simulink model "sampleModel1895"  (R2023a)
settings: Solver=VariableStepAuto  StartTime=0.0  StopTime=10.0  RelTol=1e-3
libraries: hdlsllib x3, simulink x1
settings Model: Creator=user1  LastModifiedBy=user1

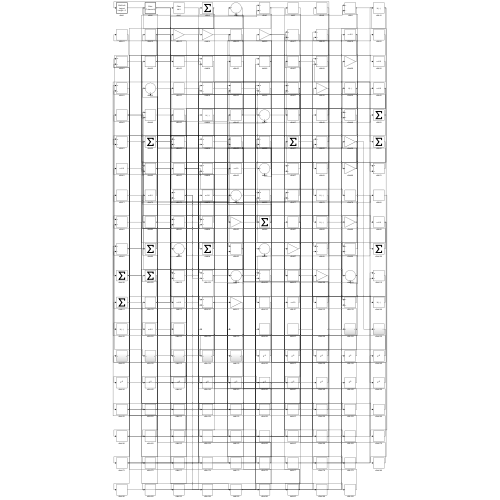
[thumbnail: Simulink's stored preview of the top-level diagram]
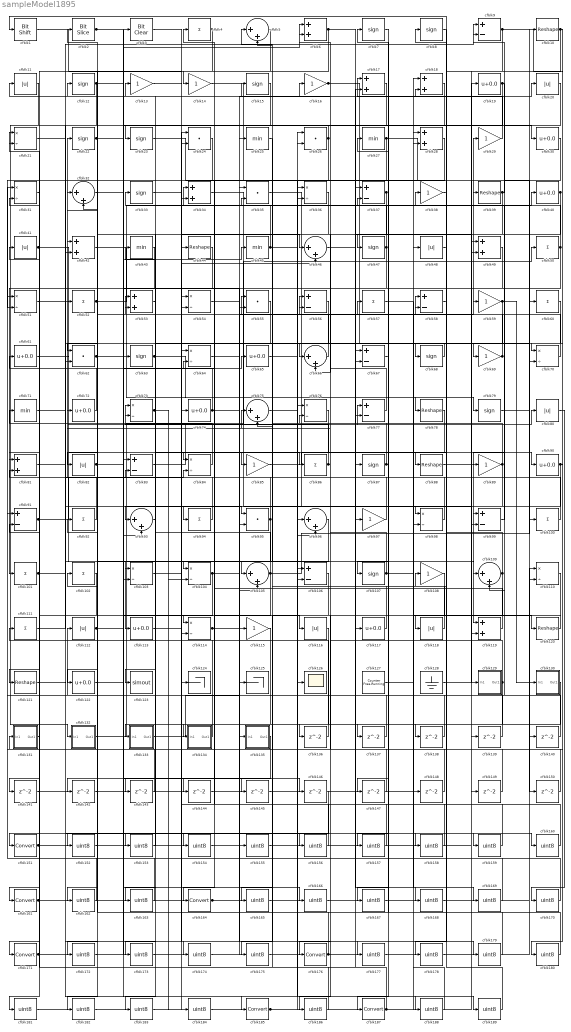
== system sampleModel1895 ==
  cfblk1 : hdlsllib/Logic and Bit Operations/Bit Shift  mode=Shift Left Logical  N=0
  cfblk{10,39,44,78,88,120..121} (7 alike) : Reshape
  cfblk{4,50,52,57,60,86,92,94,100..102,111} (12 alike) : Sum  Inputs=+
  cfblk{21,31,36,51,54,64,70,73,76,84,98,103..104,110,114} (15 alike) : Product  Inputs=*/  RndMeth=Zero  SaturateOnIntegerOverflow=on
  cfblk{5,32,46,66,75,93,96,105,109} (9 alike) : Sum  Inputs=|++
  cfblk{9,37,56,58,67,77,83,91,99,106} (10 alike) : Sum  Inputs=+-
  cfblk{7..8,12,15,22..23,33,47,63,68,79,87,107} (13 alike) : Signum
  cfblk{13..14,16,29,38,59,69,85,89,97,108,115} (12 alike) : Gain
  cfblk{11,20,41,48,80,82,112,116,118} (9 alike) : Abs  SaturateOnIntegerOverflow=off
  cfblk{19,30,40,61,65,72,74,90,113,117,122} (11 alike) : Bias  Bias=0.0  SaturateOnIntegerOverflow=off
  cfblk{6,17..18,28,34,42,49,53,81,119} (10 alike) : Sum
  cfblk123 : ToWorkspace  VariableName=simout  SaveFormat=Timeseries  SampleTime=-1
  cfblk124 : Terminator
  cfblk125 : Terminator
  cfblk126 : Scope
  cfblk127 : hdlsllib/Sources/Counter Free-Running  NumBits=16  tsamp=-1
  cfblk128 : Ground
  cfblk129 : Subsystem
      settings: LibrarySourceBlock=|
      | hdlsllib/Ports &
      | Subsystems/Subsystem
  cfblk130 : Subsystem
      settings: LibrarySourceBlock=|
      | hdlsllib/Ports &
      | Subsystems/Subsystem
  cfblk131 : Subsystem
      settings: LibrarySourceBlock=|
      | hdlsllib/Ports &
      | Subsystems/Subsystem
  cfblk132 : Subsystem
      settings: LibrarySourceBlock=|
      | hdlsllib/Ports &
      | Subsystems/Subsystem
  cfblk133 : Subsystem
      settings: LibrarySourceBlock=|
      | hdlsllib/Ports &
      | Subsystems/Subsystem
  cfblk134 : Subsystem
      settings: LibrarySourceBlock=|
      | hdlsllib/Ports &
      | Subsystems/Subsystem
  cfblk135 : Subsystem
      settings: LibrarySourceBlock=|
      | hdlsllib/Ports &
      | Subsystems/Subsystem
  cfblk{136..150} (15 alike) : Delay  SampleTime=1
  cfblk{151,161,164,171,176,185,187} (7 alike) : DataTypeConversion  SaturateOnIntegerOverflow=off  RndMeth=Floor
  cfblk{152..160,162..163,165..170,172..175,177..184,186,188..189} (32 alike) : DataTypeConversion  OutDataTypeStr=uint8  SaturateOnIntegerOverflow=off  RndMeth=Floor
  cfblk2 : hdlsllib/Logic and Bit Operations/Bit Slice  lidx=7  ridx=0
  cfblk{24,26,35,55,62,95} (6 alike) : DotProduct  OutDataTypeStr=Inherit: Inherit via internal rule
  cfblk{25,27,43,45,71} (5 alike) : MinMax
  cfblk3 : simulink/Logic and Bit Operations/Bit Clear  iBit=0
      settings: LibrarySourceBlock=|
      | hdlsllib/Logic and Bit
      | Operations/Bit Clear
  wires:
  cfblk51/1 -> cfblk77/1
  cfblk109/1 -> cfblk58/2, cfblk165/1
  cfblk11/1 -> cfblk132/1(In1)
  cfblk48/1 -> cfblk1/1
  cfblk8/1 -> cfblk88/1
  cfblk88/1 -> cfblk119/1
  cfblk49/1 -> cfblk101/1
  cfblk28/1 -> cfblk164/1
  cfblk94/1 -> cfblk22/1
  cfblk26/1 -> cfblk23/1, cfblk94/1
  cfblk114/1 -> cfblk59/1, cfblk144/1
  cfblk59/1 -> cfblk107/1, cfblk130/1(In1)
  cfblk20/1 -> cfblk112/1
  cfblk119/1 -> cfblk34/1
  cfblk16/1 -> cfblk68/1, cfblk79/1
  cfblk9/1 -> cfblk70/1, cfblk119/2
  cfblk44/1 -> cfblk171/1
  cfblk35/1 -> cfblk129/1(In1)
  cfblk31/1 -> cfblk161/1
  cfblk60/1 -> cfblk69/1
  cfblk4/1 -> cfblk81/1, cfblk14/1
  cfblk105/1 -> cfblk10/1, cfblk53/1, cfblk154/1
  cfblk86/1 -> cfblk73/1, cfblk6/1
  cfblk72/1 -> cfblk42/1
  cfblk22/1 -> cfblk30/1, cfblk6/2
  cfblk132/1(Out1) -> cfblk50/1
  cfblk42/1 -> cfblk126/1
  cfblk23/1 -> cfblk100/1
  cfblk68/1 -> cfblk66/1
  cfblk55/1 -> cfblk104/1
  cfblk84/1 -> cfblk61/1
  cfblk29/1 -> cfblk17/1
  cfblk18/1 -> cfblk187/1
  cfblk14/1 -> cfblk76/1
  cfblk71/1 -> cfblk185/1
  cfblk69/1 -> cfblk8/1, cfblk2/1
  cfblk112/1 -> cfblk63/1, cfblk45/1
  cfblk70/1 -> cfblk29/1
  cfblk90/1 -> cfblk131/1(In1), cfblk109/2
  cfblk34/1 -> cfblk98/1
  cfblk133/1(Out1) -> cfblk25/1
  cfblk91/1 -> cfblk83/2, cfblk84/2
  cfblk40/1 -> cfblk67/2, cfblk103/1
  cfblk25/1 -> cfblk85/1
  cfblk102/1 -> cfblk151/1
  cfblk116/1 -> cfblk134/1(In1)
  cfblk63/1 -> cfblk78/1, cfblk46/2, cfblk40/1
  cfblk67/1 -> cfblk27/1
  cfblk99/1 -> cfblk39/1
  cfblk113/1 -> cfblk34/2
  cfblk101/1 -> cfblk106/2, cfblk159/1
  cfblk37/1 -> cfblk66/2, cfblk152/1
  cfblk19/1 -> cfblk99/1, cfblk62/2
  cfblk104/1 -> cfblk122/1, cfblk146/1
  cfblk85/1 -> cfblk90/1
  cfblk83/1 -> cfblk20/1
  cfblk120/1 -> cfblk118/1
  cfblk45/1 -> cfblk33/1, cfblk189/1
  cfblk52/1 -> cfblk17/2, cfblk135/1(In1)
  cfblk41/1 -> cfblk84/1, cfblk95/1
  cfblk87/1 -> cfblk53/2, cfblk137/1
  cfblk82/1 -> cfblk32/2, cfblk65/1
  cfblk2/1 -> cfblk55/2, cfblk188/1
  cfblk32/1 -> cfblk116/1
  cfblk61/1 -> cfblk113/1
  cfblk65/1 -> cfblk109/1
  cfblk66/1 -> cfblk12/1
  cfblk76/1 -> cfblk105/1
  cfblk74/1 -> cfblk21/1, cfblk58/1
  cfblk10/1 -> cfblk178/1, cfblk180/1
  cfblk30/1 -> cfblk89/1
  cfblk50/1 -> cfblk4/1, cfblk103/2
  cfblk95/1 -> cfblk133/1(In1), cfblk43/1
  cfblk100/1 -> cfblk5/1
  cfblk134/1(Out1) -> cfblk91/2
  cfblk21/1 -> cfblk70/2
  cfblk127/1 -> cfblk48/1
  cfblk7/1 -> cfblk47/1
  cfblk1/1 -> cfblk24/2
  cfblk62/1 -> cfblk114/1, cfblk93/2
  cfblk118/1 -> cfblk73/2
  cfblk17/1 -> cfblk121/1
  cfblk33/1 -> cfblk46/1
  cfblk103/1 -> cfblk80/1
  cfblk97/1 -> cfblk52/1
  cfblk47/1 -> cfblk35/2, cfblk82/1
  cfblk98/1 -> cfblk15/1
  cfblk58/1 -> cfblk38/1
  cfblk12/1 -> cfblk42/2, cfblk86/1, cfblk166/1
  cfblk73/1 -> cfblk104/2, cfblk184/1
  cfblk111/1 -> cfblk9/1
  cfblk39/1 -> cfblk9/2, cfblk147/1
  cfblk117/1 -> cfblk55/1
  cfblk89/1 -> cfblk93/1, cfblk56/2
  cfblk92/1 -> cfblk81/2
  cfblk77/1 -> cfblk11/1
  cfblk110/1 -> cfblk176/1
  cfblk107/1 -> cfblk120/1, cfblk72/1, cfblk157/1
  cfblk128/1 -> cfblk49/1
  cfblk131/1(Out1) -> cfblk111/1
  cfblk129/1(Out1) -> cfblk56/1, cfblk136/1
  cfblk27/1 -> cfblk60/1, cfblk114/2
  cfblk24/1 -> cfblk51/2
  cfblk6/1 -> cfblk49/2, cfblk62/1
  cfblk53/1 -> cfblk123/1
  cfblk136/1 -> cfblk21/2
  cfblk137/1 -> cfblk24/1
  cfblk38/1 -> cfblk138/1
  cfblk138/1 -> cfblk51/1
  cfblk139/1 -> cfblk32/1
  cfblk140/1 -> cfblk83/1
  cfblk15/1 -> cfblk141/1
  cfblk141/1 -> cfblk98/2
  cfblk5/1 -> cfblk142/1
  cfblk142/1 -> cfblk105/2
  cfblk93/1 -> cfblk143/1
  cfblk143/1 -> cfblk91/1
  cfblk144/1 -> cfblk67/1
  cfblk122/1 -> cfblk145/1
  cfblk145/1 -> cfblk77/2
  cfblk147/1 -> cfblk76/2
  cfblk148/1 -> cfblk26/1
  cfblk149/1 -> cfblk37/2
  cfblk79/1 -> cfblk150/1
  cfblk150/1 -> cfblk16/1
  cfblk151/1 -> cfblk19/1, cfblk26/2
  cfblk152/1 -> cfblk102/1
  cfblk115/1 -> cfblk153/1
  cfblk153/1 -> cfblk13/1
  cfblk154/1 -> cfblk115/1
  cfblk64/1 -> cfblk155/1
  cfblk155/1 -> cfblk97/1
  cfblk13/1 -> cfblk156/1
  cfblk156/1 -> cfblk64/1
  cfblk157/1 -> cfblk64/2
  cfblk75/1 -> cfblk158/1
  cfblk158/1 -> cfblk35/1
  cfblk159/1 -> cfblk75/1
  cfblk121/1 -> cfblk160/1
  cfblk160/1 -> cfblk75/2
  cfblk161/1 -> cfblk87/1, cfblk124/1
  cfblk43/1 -> cfblk162/1
  cfblk162/1 -> cfblk31/1
  cfblk56/1 -> cfblk163/1
  cfblk163/1 -> cfblk31/2
  cfblk164/1 -> cfblk125/1, cfblk117/1
  cfblk165/1 -> cfblk28/1
  cfblk166/1 -> cfblk28/2
  cfblk108/1 -> cfblk167/1
  cfblk167/1 -> cfblk140/1
  cfblk46/1 -> cfblk168/1
  cfblk168/1 -> cfblk108/1
  cfblk57/1 -> cfblk169/1
  cfblk169/1 -> cfblk41/1
  cfblk80/1 -> cfblk170/1
  cfblk170/1 -> cfblk57/1
  cfblk171/1 -> cfblk95/2, cfblk99/2, cfblk3/1
  cfblk135/1(Out1) -> cfblk172/1
  cfblk172/1 -> cfblk44/1
  cfblk36/1 -> cfblk173/1
  cfblk173/1 -> cfblk74/1
  cfblk81/1 -> cfblk174/1
  cfblk174/1 -> cfblk36/1
  cfblk106/1 -> cfblk175/1
  cfblk175/1 -> cfblk36/2
  cfblk176/1 -> cfblk106/1, cfblk92/1
  cfblk3/1 -> cfblk177/1
  cfblk177/1 -> cfblk110/1
  cfblk178/1 -> cfblk110/2
  cfblk54/1 -> cfblk179/1
  cfblk179/1 -> cfblk7/1
  cfblk180/1 -> cfblk54/1
  cfblk146/1 -> cfblk181/1
  cfblk181/1 -> cfblk54/2
  cfblk96/1 -> cfblk182/1
  cfblk182/1 -> cfblk139/1
  cfblk78/1 -> cfblk183/1
  cfblk183/1 -> cfblk96/1
  cfblk184/1 -> cfblk96/2
  cfblk185/1 -> cfblk149/1, cfblk148/1
  cfblk130/1(Out1) -> cfblk186/1
  cfblk186/1 -> cfblk71/1
  cfblk187/1 -> cfblk5/2, cfblk37/1
  cfblk188/1 -> cfblk18/1
  cfblk189/1 -> cfblk18/2

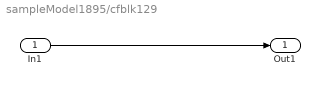
== system sampleModel1895/cfblk129 ==
  In1 : Inport
  Out1 : Outport
  wires:
  In1/1 -> Out1/1

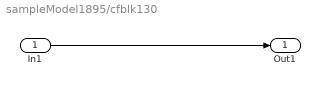
== system sampleModel1895/cfblk130 ==
  In1 : Inport
  Out1 : Outport
  wires:
  In1/1 -> Out1/1

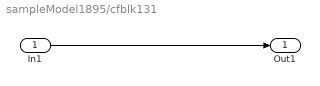
== system sampleModel1895/cfblk131 ==
  In1 : Inport
  Out1 : Outport
  wires:
  In1/1 -> Out1/1

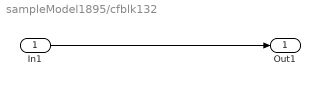
== system sampleModel1895/cfblk132 ==
  In1 : Inport
  Out1 : Outport
  wires:
  In1/1 -> Out1/1

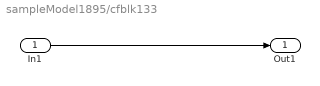
== system sampleModel1895/cfblk133 ==
  In1 : Inport
  Out1 : Outport
  wires:
  In1/1 -> Out1/1

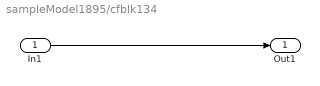
== system sampleModel1895/cfblk134 ==
  In1 : Inport
  Out1 : Outport
  wires:
  In1/1 -> Out1/1

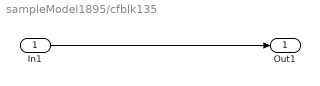
== system sampleModel1895/cfblk135 ==
  In1 : Inport
  Out1 : Outport
  wires:
  In1/1 -> Out1/1
